simulink model "FM_modul"  (R2020a)
settings: Solver=VariableStepAuto  StartTime=0.0  StopTime=50  RelTol=1e-3
settings Model: Creator=Atharv Sharma  LastModifiedBy=Atharv Sharma

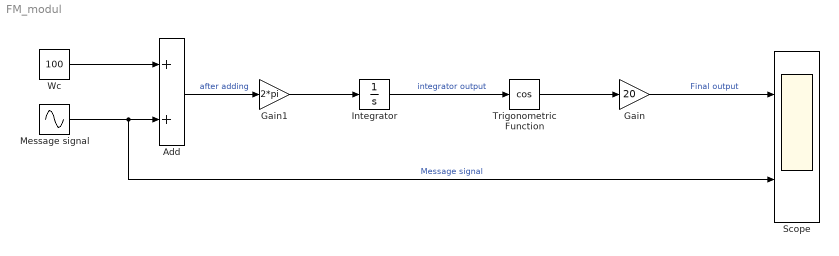
== system FM_modul ==
  Add : Sum
  Gain : Gain  Gain=20
  Gain1 : Gain  Gain=2*pi
  Integrator : Integrator
  Message signal : Sin  Amplitude=30  Frequency=2*pi*10  SampleTime=.0001
  Scope : Scope  NumInputPorts=2
  Trigonometric Function : Trigonometry  Operator=cos
  Wc : Constant  Value=100  SampleTime=.0001
  wires:
  Trigonometric Function/1 -> Gain/1
  Add/1 -> Gain1/1  "after adding"
  Message signal/1 -> Scope/2, Add/2  "Message signal"
  Wc/1 -> Add/1
  Integrator/1 -> Trigonometric Function/1  "integrator output"
  Gain/1 -> Scope/1  "Final output"
  Gain1/1 -> Integrator/1
